simulink model "test"  (R2023b)
settings: Solver=VariableStepAuto  StartTime=0.0  StopTime=10.0  RelTol=1e-6
settings Model: Creator=jefft  LastModifiedBy=jefft
settings SFSimCC: SimCustomHeaderCode="#include \"function.h\""  SimUserSources=function.cpp  SimUserIncludeDirs=ASTRAFlightSoftware/lib/math  SimTargetLang=C++

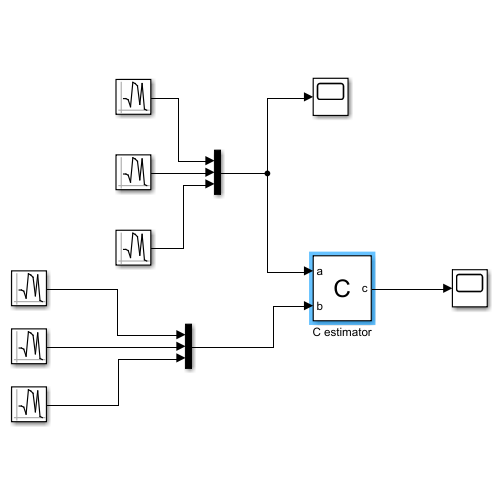
[thumbnail: Simulink's stored preview of the top-level diagram]
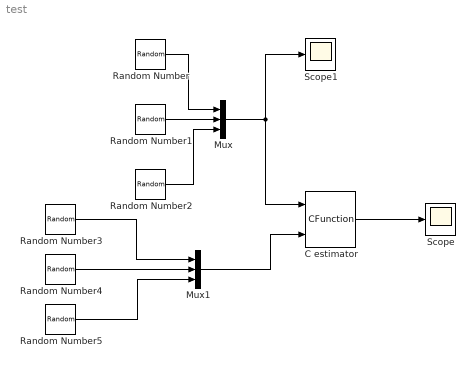
== system test ==
  C estimator : CFunction  OutputCode=|
      | // testVectors(i, o)
      | addVectors(a, b, c);
  Mux : Mux  Inputs=3
  Mux1 : Mux  Inputs=3
  Random Number : RandomNumber  Mean=1  Seed=1  SampleTime=0.1
  Random Number1 : RandomNumber  Mean=1  Seed=2  SampleTime=0.1
  Random Number2 : RandomNumber  Mean=1  Seed=5  SampleTime=0.1
  Random Number3 : RandomNumber  Mean=1  Seed=1  SampleTime=0.1
  Random Number4 : RandomNumber  Mean=1  SampleTime=0.1
  Random Number5 : RandomNumber  Mean=1  Seed=6  SampleTime=0.1
  Scope : Scope
  Scope1 : Scope
  wires:
  Mux/1 -> C estimator/1, Scope1/1
  Random Number/1 -> Mux/1
  C estimator/1 -> Scope/1
  Random Number1/1 -> Mux/2
  Random Number2/1 -> Mux/3
  Random Number5/1 -> Mux1/3
  Mux1/1 -> C estimator/2
  Random Number4/1 -> Mux1/2
  Random Number3/1 -> Mux1/1
